simulink model "qpsk_tx"  (Simulink 7.9)
settings: Solver=FixedStepDiscrete  SolverMode=SingleTasking  StartTime=0.0  StopTime=4e-5  RelTol=1e-3
PreLoadFcn:
  | qpsk_syn_init;
undefined symbols (not defined in the file): Fs, get, qpsk_syn_params, sided, Two
libraries: shlslibv1 x16, commsink2 x3, dspsnks4 x2, commrandsrc2 x1
settings Model: synDspstartup=OK  Creator=sszilvasi  LastModifiedBy=sszilvasi
settings DataIOCC: SaveOutput=off  SignalLogging=off  SaveTime=off
settings OptimizationCC: InlineParams=on
settings DebuggingCC: AlgebraicLoopMsg=error  InheritedTsInSrcMsg=none

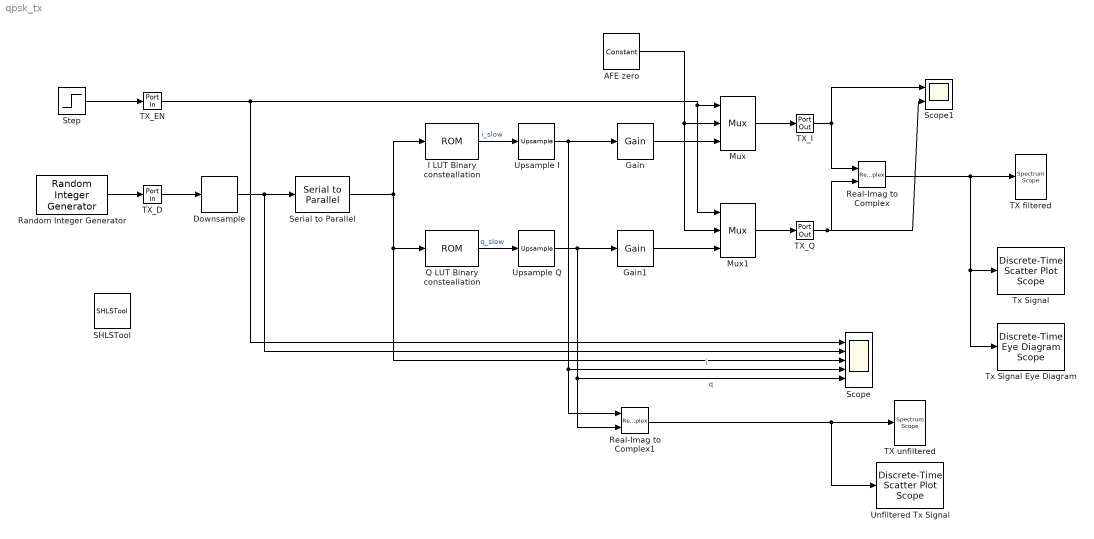
== system qpsk_tx ==
  AFE zero : shlslibv1/Sources/Constant  syn_cst_val=0  syn_cst_fl=9  syn_cst_dt=signed  syn_cst_rnd=on  syn_cst_st=-1  synBlockType=primitive  synLatency=0  synBlockId=15
  Downsample : shlslibv1/Signal Operations/Downsample  syn_r_val=qpsk_syn_params.CL/qpsk_syn_params.bps  syn_sample_offset=2  syn_sync_mode=No Sync  synBlockType=primitive  synLatency=1  synBlockId=7
  Gain : shlslibv1/Math Functions/Gain  syn_gain_val=.5  syn_gain_fl=8  syn_gain_dt=signed  syn_gain_rnd=on  syn_out_f=Full Precision  syn_out_wl=16  syn_out_fl=8  syn_out_dt=signed  syn_out_sat=off  syn_out_rnd=Floor (Truncate)  synBlockType=primitive  synLatency=0  synBlockId=3  syn_opr_mode=0
  Gain1 : shlslibv1/Math Functions/Gain  syn_gain_val=.5  syn_gain_fl=8  syn_gain_dt=signed  syn_gain_rnd=on  syn_out_f=Full Precision  syn_out_wl=16  syn_out_fl=8  syn_out_dt=signed  syn_out_sat=off  syn_out_rnd=Floor (Truncate)  synBlockType=primitive  synLatency=0  synBlockId=3  syn_opr_mode=0
  "I LUT Binary consteallation " : shlslibv1/Memories/ROM  syn_rom_vec=[1 -1 -1 1]  syn_out_wl=2  syn_out_fl=0  syn_out_dt=signed  syn_out_sat=off  syn_out_rnd=on  synBlockType=primitive  synLatency=1  synBlockId=62
  Mux : shlslibv1/Signal Operations/Mux  syn_in_nb=2  syn_out_f=Full Precision  syn_out_wl=16  syn_out_fl=8  syn_out_dt=signed  synBlockType=primitive  synLatency=0  synBlockId=16
  Mux1 : shlslibv1/Signal Operations/Mux  syn_in_nb=2  syn_out_f=Full Precision  syn_out_wl=16  syn_out_fl=8  syn_out_dt=signed  synBlockType=primitive  synLatency=0  synBlockId=16
  Q LUT Binary consteallation : shlslibv1/Memories/ROM  syn_rom_vec=[1 1 -1 -1]  syn_out_wl=2  syn_out_fl=0  syn_out_dt=signed  syn_out_sat=off  syn_out_rnd=on  synBlockType=primitive  synLatency=1  synBlockId=62
  Random Integer Generator : commrandsrc2/Random Integer Generator  mul=2  seed=37  Ts=qpsk_syn_params.Tc/qpsk_syn_params.bps  frameBased=off  sampPerFrame=1  orient=off  outDataType=double
  Real-Imag to Complex : RealImagToComplex
  Real-Imag to Complex1 : RealImagToComplex
  SHLSTool : shlslibv1/SHLSTool  synBlockType=tool  syn_dsp_mode=FPGA
  Scope : Scope  NumInputPorts=5
      settings: YMin=-5~-5~-5~-5~-5  YMax=5~5~5~5~5
  Scope1 : Scope  NumInputPorts=2
      settings: YMin=-5~-5  YMax=5~5
  Serial to Parallel : shlslibv1/Signal Operations/Serial to Parallel  syn_pack_nb=2  syn_pack_ord=LSB to MSB  syn_out_f=Automatic  syn_out_wl=17  syn_out_fl=9  syn_out_dt=signed  synBlockType=custom  synLatency=1
  Step : Step  Time=qpsk_syn_params.Tc/qpsk_syn_params.bps*5  SampleTime=qpsk_syn_params.Tc
  TX filtered : dspsnks4/Spectrum Scope  ScopeProperties=on  Domain=Frequency  HorizSpan=1  UseBuffer=on  BufferSize=128  Overlap=0  TreatMby1Signals=One channel  inpFftLenInherit=off  FFTlength=128  numAvg=2  DisplayProperties=off  AxisGrid=on  Memory=off  FrameNumber=on  AxisLegend=off  AxisZoom=off  OpenScopeAtSimStart=off  OpenScopeImmediately=off  FigPos=get(0,'defaultfigureposition')  AxisProperties=off  XUnits=Hertz  XRange=Two-sided ((-Fs/2...Fs/2])  XDisplay=0  InheritXIncr=on  XIncr=1.0  XLabel=Samples  XLimit=Auto  YUnits=dBW/Hertz  XMax=1  XMin=0  YLabel=Magnitude-squared, dB  LineProperties=off  wintypeSpecScope=Hann  RsSpecScope=50  betaSpecScope=5  winsampSpecScope=Periodic  XAxisParamsVer=6.9  isFrameUpgraded=on
      settings: YMin=-10  YMax=10
  TX unfiltered : dspsnks4/Spectrum Scope  ScopeProperties=on  Domain=Frequency  HorizSpan=1  UseBuffer=on  BufferSize=128  Overlap=0  TreatMby1Signals=One channel  inpFftLenInherit=off  FFTlength=128  numAvg=2  DisplayProperties=off  AxisGrid=on  Memory=off  FrameNumber=on  AxisLegend=off  AxisZoom=off  OpenScopeAtSimStart=off  OpenScopeImmediately=off  FigPos=get(0,'defaultfigureposition')  AxisProperties=off  XUnits=Hertz  XRange=Two-sided ((-Fs/2...Fs/2])  XDisplay=0  InheritXIncr=on  XIncr=1.0  XLabel=Samples  XLimit=Auto  YUnits=dBW/Hertz  XMax=1  XMin=0  YLabel=Magnitude-squared, dB  LineProperties=off  wintypeSpecScope=Hann  RsSpecScope=50  betaSpecScope=5  winsampSpecScope=Periodic  XAxisParamsVer=6.9  isFrameUpgraded=on
      settings: YMin=-10  YMax=10
  TX_D : shlslibv1/Ports & Subsystems/Port In  syn_out_wl=1  syn_out_fl=0  syn_out_dt=unsigned  syn_out_st=qpsk_syn_params.Ts  syn_capture=off  syn_register=on  syn_out_sat=off  syn_out_rnd=on  synBlockType=port  synLatency=1  synBlockId=0
  TX_EN : shlslibv1/Ports & Subsystems/Port In  syn_out_wl=1  syn_out_fl=0  syn_out_dt=unsigned  syn_out_st=qpsk_syn_params.Ts  syn_capture=on  syn_register=on  syn_out_sat=off  syn_out_rnd=on  synBlockType=port  synLatency=1  synBlockId=0
  TX_I : shlslibv1/Ports & Subsystems/Port Out  syn_capture=off  syn_register=off  synBlockType=port  synLatency=0  synBlockId=1
  TX_Q : shlslibv1/Ports & Subsystems/Port Out  syn_capture=off  syn_register=off  synBlockType=port  synLatency=0  synBlockId=1
  Tx Signal : commsink2/Discrete-Time Scatter Plot Scope  Tag=ScatterPlot  sampPerSymb=qpsk_syn_params.CL  offsetEye=4  numTraces=200  numNewFrames=40  LineMarkers=.  LineColors=b  fading=on  render=on  AxisGrid=on  xMin=-1.05  xMax=1.05  yMin=-1.05  yMax=1.05  inphaseLabel=In-phase Amplitude  quadratureLabel=Quadrature Amplitude  openScopeAtSimStart=off  FrameNumber=off  FigPos=get(0,'defaultfigureposition');  figTitle=Scatter Plot  numLinesMax=8  block_type_=scatter
  Tx Signal Eye Diagram : commsink2/Discrete-Time Eye Diagram Scope  Tag=EyeDiagram  sampPerSymb=8  offsetEye=0  symbPerTrace=1  numTraces=40  numNewFrames=10  LineStyles=-  LineColors=b  dupPoints=on  fading=on  render=on  AxisGrid=on  yMin=-18.129248046875  yMax=6.77067138671875  inphaseLabel=In-phase Amplitude  quadratureLabel=Quadrature Amplitude  openScopeAtSimStart=off  dispDiagram=In-phase and Quadrature  FrameNumber=off  FigPos=get(0,'defaultfigureposition');  figTitle=Eye Diagram  block_type_=eye  numLinesMax=8
  Unfiltered Tx Signal : commsink2/Discrete-Time Scatter Plot Scope  Tag=ScatterPlot  sampPerSymb=qpsk_syn_params.CL  offsetEye=4  numTraces=200  numNewFrames=40  LineMarkers=.  LineColors=b  fading=on  render=on  AxisGrid=on  xMin=-1.05  xMax=1.05  yMin=-1.05  yMax=1.05  inphaseLabel=In-phase Amplitude  quadratureLabel=Quadrature Amplitude  openScopeAtSimStart=off  FrameNumber=off  FigPos=get(0,'defaultfigureposition');  figTitle=Scatter Plot  numLinesMax=8  block_type_=scatter
  Upsample I : shlslibv1/Signal Operations/Upsample  syn_r_val=qpsk_syn_params.CL  syn_in_hold=on  syn_sample_offset=0  syn_sync_mode=No Sync  synBlockType=primitive  synLatency=0  synBlockId=6
  Upsample Q : shlslibv1/Signal Operations/Upsample  syn_r_val=qpsk_syn_params.CL  syn_in_hold=on  syn_sample_offset=0  syn_sync_mode=No Sync  synBlockType=primitive  synLatency=0  synBlockId=6
  wires:
  TX_D/1 -> Downsample/1
  Q LUT Binary consteallation/1 -> Upsample Q/1  "q_slow"
  "I LUT Binary consteallation "/1 -> Upsample I/1  "i_slow"
  Random Integer Generator/1 -> TX_D/1
  Real-Imag to Complex/1 -> TX filtered/1, Tx Signal Eye Diagram/1, Tx Signal/1
  TX_I/1 -> Real-Imag to Complex/1, Scope1/1
  TX_Q/1 -> Real-Imag to Complex/2, Scope1/2
  Real-Imag to Complex1/1 -> TX unfiltered/1, Unfiltered Tx Signal/1
  Step/1 -> TX_EN/1
  Mux/1 -> TX_I/1
  TX_EN/1 -> Mux/1, Mux1/1, Scope/1
  AFE zero/1 -> Mux/2, Mux1/2
  Mux1/1 -> TX_Q/1
  Downsample/1 -> Serial to Parallel/1, Scope/2
  Upsample Q/1 -> Real-Imag to Complex1/2, Scope/5, Gain1/1  "q"
  Upsample I/1 -> Real-Imag to Complex1/1, Scope/4, Gain/1  "i"
  Gain/1 -> Mux/3
  Gain1/1 -> Mux1/3
  Serial to Parallel/1 -> "I LUT Binary consteallation "/1, Q LUT Binary consteallation/1, Scope/3
